simulink model "ev3_gyroboy_remote_control"  (R2021b)
settings: Solver=FixedStepDiscrete  StartTime=0.0  StopTime=inf  FixedStep=0.15  RelTol=1e-3
libraries: androiduilib x3, androidsensorlib x1, androidcommunicationlib x1
settings Model: Creator=The MathWorks, Inc.
settings SolverCC: AlgebraicLoopSolver=TrustRegion  PositivePriorityOrder=on
settings DataIOCC: ReturnWorkspaceOutputs=off
settings OptimizationCC: MaxStackSize=64
settings DebuggingCC: ParameterPrecisionLossMsg=none  ParameterTunabilityLossMsg=error  ArithmeticOperatorsInVariantConditions=warning
settings HardwareCC: ProdBitPerPointer=32  ProdBitPerSizeT=32  ProdBitPerPtrDiffT=32  ProdLargestAtomicInteger=Long  ProdLargestAtomicFloat=Double  ProdWordSize=32  ProdHWDeviceType=ARM Compatible->ARM Cortex  UseEmbeddedCoderFeatures=off  UseSimulinkCoderFeatures=off
settings SFSimCC: SimUseLocalCustomCode=off  CustomCodeUndefinedFunction=UseInterfaceOnly
settings RTWCC: Description=Embedded Coder  SystemTargetFile=ert.tlc  HardwareBoard=Android Device  TLCOptions="-aInlineSetEventsForThisBaseRateFcn=TLC_FALSE -aSuppressMultiTaskScheduler=TLC_FALSE  -aRateBasedStepFcn=0"  TemplateMakefile=ert_default_tmf  GenerateReport=on  RTWUseLocalCustomCode=off  Toolchain=Android SDK/NDK Tools  LaunchReport=on  DLArmComputeVersion=20.02.1
settings CodeAppCC: ForceParamTrailComments=on  OperatorAnnotations=on  StateflowObjectComments=on  MATLABSourceComments=on
settings ERTTargetCC: ERTCustomFileBanners=off  SupportContinuousTime=on  SupportNonInlinedSFcns=on  RemoveResetFunc=off  SupportVariableSizeSignals=on  ModelStepFunctionPrototypeControlCompliant=off
settings ConfigComp: CovMetricSettings=dswe  CovBoundaryAbsTol=1.0e-5
settings SettingsController: UseSoCProfilerForTargets=0

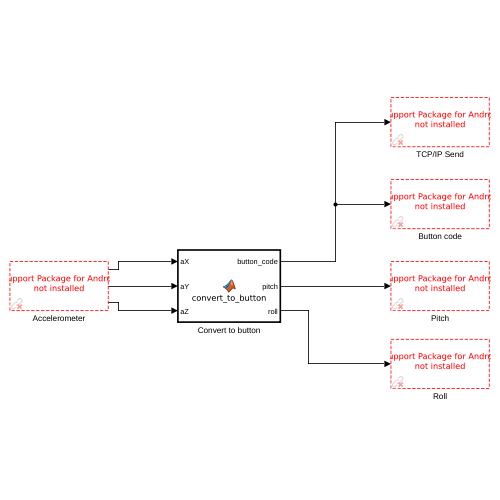
[thumbnail: Simulink's stored preview of the top-level diagram]
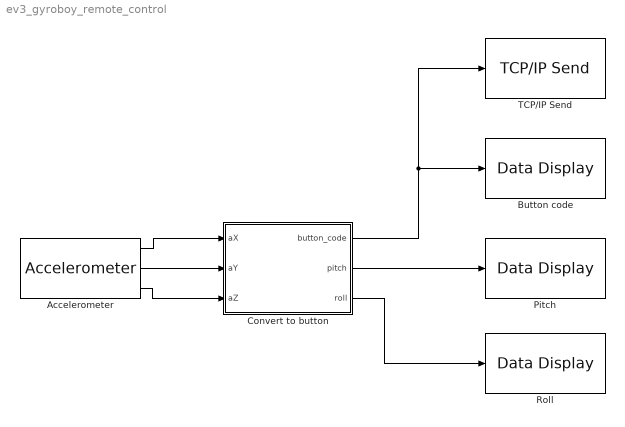
== system ev3_gyroboy_remote_control ==
  Accelerometer : androidsensorlib/Accelerometer  OutputVector=off  SampleTime=0.15  BlockPlatform=Android
      settings: SourceProductName=Simulink Support Package for Android Devices
  Button code : androiduilib/Data Display  DataDisplayId=ev3_gyroboy_remote_control/Button_code  Format=Integer  Precision=1  SimulateUsing=Code generation  blockPlatform=Android
      settings: SourceProductName=Simulink Support Package for Android Devices
  Convert to button : MATLAB Function  TreatAsAtomicUnit=on
  Pitch : androiduilib/Data Display  DataDisplayId=ev3_gyroboy_remote_control/Pitch  Format=Float  Precision=1  SimulateUsing=Code generation  blockPlatform=Android
      settings: SourceProductName=Simulink Support Package for Android Devices
  Roll : androiduilib/Data Display  DataDisplayId=ev3_gyroboy_remote_control/Roll  Format=Float  Precision=1  SimulateUsing=Code generation  blockPlatform=Android
      settings: SourceProductName=Simulink Support Package for Android Devices
  TCP/IP Send : androidcommunicationlib/TCP//IP Send  TCPSendId=ev3_gyroboy_remote_control/TCP//IP_Send  Mode_=Client  LocalServerPort_=25000  RemoteAddr_=192.168.1.11  RemoteServerPort_=25000  SimulateUsing=Code generation  ClientPortBindingSelection_=off  ClientPortToBind_=35000  BlockingMode_=off  BlockTimeout_=0.1
      settings: SourceProductName=Simulink Support Package for Android Devices
  wires:
  Accelerometer/3 -> Convert to button/3(aZ)
  Accelerometer/2 -> Convert to button/2(aY)
  Accelerometer/1 -> Convert to button/1(aX)
  Convert to button/1(button_code) -> Button code/1, TCP/IP Send/1
  Convert to button/2(pitch) -> Pitch/1
  Convert to button/3(roll) -> Roll/1

== matlab function ev3_gyroboy_remote_control/Convert to button ==
  data: aX input; aY input; button_code output; aZ input; pitch output; roll output
function [button_code, pitch, roll] = convert_to_button(aX,aY,aZ)

%Convert accelerometer sensor data to roll and pitch angles.
pitch = single(180 * atan (aX/sqrt(aY*aY + aZ*aZ))/pi);
roll = single(180 * atan (aY/sqrt(aX*aX + aZ*aZ))/pi);

%This mimics EV3 IR Remote Control buttons
if (pitch>15)
    button_code =int8(3);
elseif (pitch<-15)
    button_code =int8(4);
elseif (roll>15)
    button_code =int8(2);
elseif (roll<-15)
    button_code =int8(1);
else
    button_code =int8(0);
end

end
